simulink library "mdderslib_vehicle"  (Simulink 7.8)
settings: Solver=ode45  StartTime=0.0  StopTime=10.0  RelTol=1e-3
undefined symbols (not defined in the file or in its folder): S, VC
libraries: simulink_extras x2, simulink x1
settings Model: Creator=bures  LastModifiedBy=bures

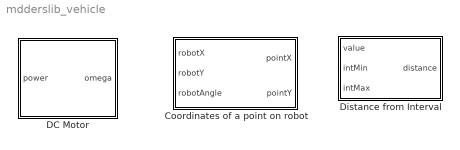
== system mdderslib_vehicle ==
  Coordinates of a point on robot : Subsystem  mask{point=S.colorSensor}
  DC Motor : Subsystem  mask{P=VC.motorL}
      mask prompts: P "Motor profile"
      mask Display:
      | port_label('input', 1, 'power');
      | port_label('output', 1, 'ticks/s');
  Distance from Interval : Subsystem
      mask Display:
      | disp('');
      | port_label('input', 1, 'value');
      | port_label('output', 1, 'distance');
      | port_label('input', 2, 'min');
      | port_label('input', 3, 'max');

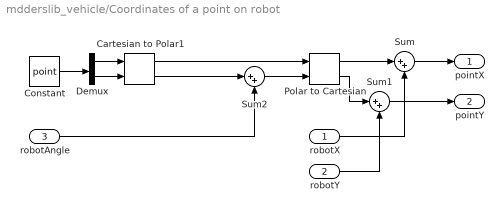
== system mdderslib_vehicle/Coordinates of a point on robot ==
  robotX : Inport
  robotY : Inport  Port=2
  robotAngle : Inport  Port=3
  Cartesian to Polar1 : simulink_extras/Transformations/Cartesian to Polar
  Constant : Constant  Value=point
  Demux : Demux  Outputs=2
  Polar to Cartesian : simulink_extras/Transformations/Polar to Cartesian
  Sum : Sum  Inputs=|++
  Sum1 : Sum  Inputs=|++
  Sum2 : Sum  Inputs=|++
  pointX : Outport
  pointY : Outport  Port=2
  wires:
  Sum1/1 -> pointY/1
  robotY/1 -> Sum1/2
  Polar to Cartesian/2 -> Sum1/1
  robotX/1 -> Sum/2
  Sum/1 -> pointX/1
  Polar to Cartesian/1 -> Sum/1
  Cartesian to Polar1/1 -> Polar to Cartesian/1
  Sum2/1 -> Polar to Cartesian/2
  robotAngle/1 -> Sum2/2
  Cartesian to Polar1/2 -> Sum2/1
  Demux/1 -> Cartesian to Polar1/1
  Demux/2 -> Cartesian to Polar1/2
  Constant/1 -> Demux/1

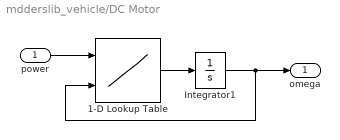
== system mdderslib_vehicle/DC Motor ==
  power : Inport
  1-D Lookup Table : Lookup_n-D  BreakpointsForDimension1=P.power  BreakpointsForDimension2=P.speed  Table=P.accel  RndMeth=Simplest  InputSameDT=on
  Integrator1 : Integrator
  omega : Outport
  wires:
  Integrator1/1 -> omega/1, 1-D Lookup Table/2
  power/1 -> 1-D Lookup Table/1
  1-D Lookup Table/1 -> Integrator1/1

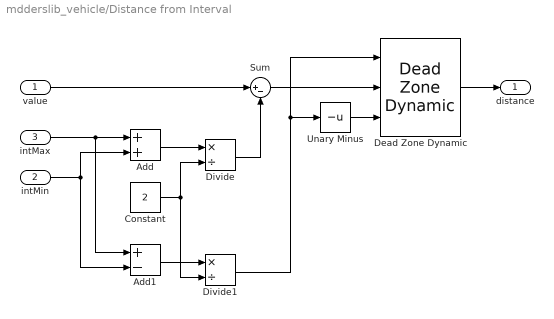
== system mdderslib_vehicle/Distance from Interval ==
  value : Inport
  intMin : Inport  Port=2
  intMax : Inport  Port=3
  Add : Sum
  Add1 : Sum  Inputs=+-
  Constant : Constant  Value=2
  Dead Zone Dynamic : simulink/Discontinuities/Dead Zone Dynamic
  Divide : Product  Inputs=*/
  Divide1 : Product  Inputs=*/
  Sum : Sum  Inputs=|+-
  Unary Minus : UnaryMinus
  distance : Outport
  wires:
  Dead Zone Dynamic/1 -> distance/1
  Unary Minus/1 -> Dead Zone Dynamic/3
  Divide1/1 -> Unary Minus/1, Dead Zone Dynamic/1
  Sum/1 -> Dead Zone Dynamic/2
  Add1/1 -> Divide1/1
  Divide/1 -> Sum/2
  value/1 -> Sum/1
  Constant/1 -> Divide1/2, Divide/2
  Add/1 -> Divide/1
  intMin/1 -> Add1/2, Add/2
  intMax/1 -> Add1/1, Add/1
